simulink model "int_crit"  (Simulink 6.4)
settings: Solver=ode45  StartTime=0.0  StopTime=10.0  RelTol=1e-3
undefined symbols (not defined in the file or in its folder): q_de, q_du, q_u
settings Model: Creator=oravec  LastModifiedBy=oravec
settings OptimizationCC: InitFltsAndDblsToZero=off
settings DebuggingCC: SignalResolutionControl=UseLocalSettings  MultiTaskDSMMsg=error  MultiTaskCondExecSysMsg=error  StrictBusMsg=ErrorLevel1
settings HardwareCC: TargetHWDeviceType=32-bit Generic

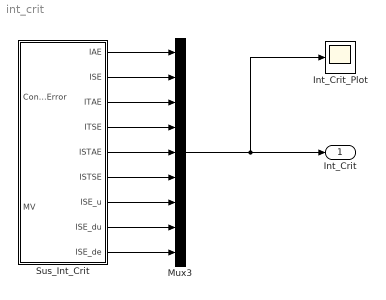
== system int_crit ==
  Int_Crit_Plot : Scope
  Mux3 : Mux  Inputs=9
  Sus_Int_Crit : Subsystem
  Int_Crit : Outport
  wires:
  Sus_Int_Crit/1(IAE) -> Mux3/1
  Sus_Int_Crit/3(ITAE) -> Mux3/3
  Sus_Int_Crit/4(ITSE) -> Mux3/4
  Sus_Int_Crit/5(ISTAE) -> Mux3/5
  Sus_Int_Crit/6(ISTSE) -> Mux3/6
  Sus_Int_Crit/7(ISE_u) -> Mux3/7
  Sus_Int_Crit/8(ISE_du) -> Mux3/8
  Sus_Int_Crit/9(ISE_de) -> Mux3/9
  Mux3/1 -> Int_Crit/1, Int_Crit_Plot/1
  Sus_Int_Crit/2(ISE) -> Mux3/2

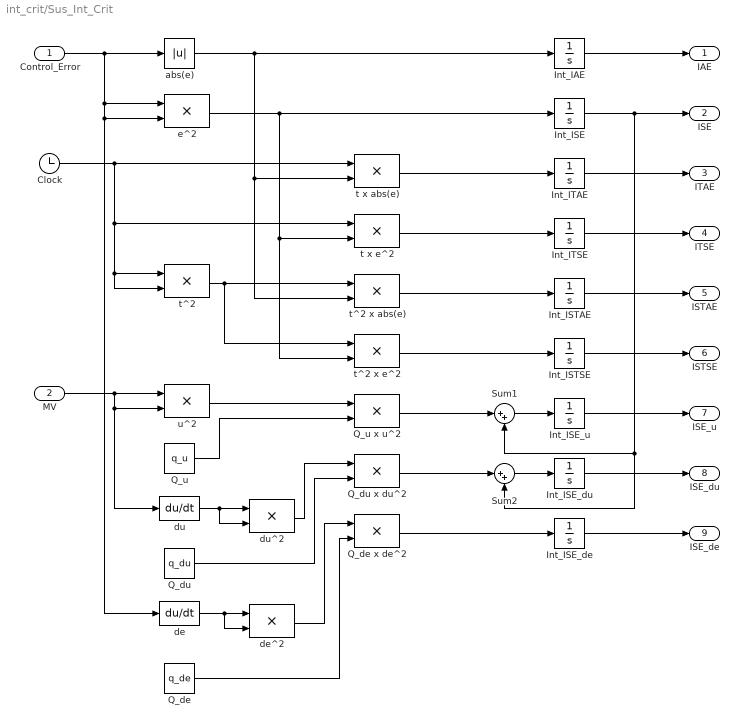
== system int_crit/Sus_Int_Crit ==
  Control_Error : Inport
  MV : Inport  Port=2
  Clock : Clock
      settings: Decimation=10
  Int_IAE : Integrator
  Int_ISE : Integrator
  Int_ISE_de : Integrator
  Int_ISE_du : Integrator
  Int_ISE_u : Integrator
  Int_ISTAE : Integrator
  Int_ISTSE : Integrator
  Int_ITAE : Integrator
  Int_ITSE : Integrator
  Q_de : Constant  Value=q_de
  Q_de x de^2 : Product  SaturateOnIntegerOverflow=on
  Q_du : Constant  Value=q_du
  Q_du x du^2 : Product  SaturateOnIntegerOverflow=on
  Q_u : Constant  Value=q_u
  Q_u x u^2 : Product  SaturateOnIntegerOverflow=on
  Sum1 : Sum  Inputs=|++  SaturateOnIntegerOverflow=on
  Sum2 : Sum  Inputs=|++  SaturateOnIntegerOverflow=on
  abs(e) : Abs  SaturateOnIntegerOverflow=on
  de : Derivative
  de^2 : Product  SaturateOnIntegerOverflow=on
  du : Derivative
  du^2 : Product  SaturateOnIntegerOverflow=on
  e^2 : Product  SaturateOnIntegerOverflow=on
  t x abs(e) : Product  SaturateOnIntegerOverflow=on
  t x e^2 : Product  SaturateOnIntegerOverflow=on
  t^2 : Product  SaturateOnIntegerOverflow=on
  t^2 x abs(e) : Product  SaturateOnIntegerOverflow=on
  t^2 x e^2 : Product  SaturateOnIntegerOverflow=on
  u^2 : Product  SaturateOnIntegerOverflow=on
  IAE : Outport
  ISE : Outport  Port=2
  ITAE : Outport  Port=3
  ITSE : Outport  Port=4
  ISTAE : Outport  Port=5
  ISTSE : Outport  Port=6
  ISE_u : Outport  Port=7
  ISE_du : Outport  Port=8
  ISE_de : Outport  Port=9
  wires:
  Control_Error/1 -> abs(e)/1, e^2/1, e^2/2, de/1
  abs(e)/1 -> Int_IAE/1, t x abs(e)/2, t^2 x abs(e)/2
  e^2/1 -> Int_ISE/1, t x e^2/2, t^2 x e^2/2
  Int_ISE/1 -> Sum1/2, Sum2/2, ISE/1
  t x abs(e)/1 -> Int_ITAE/1
  Clock/1 -> t x abs(e)/1, t x e^2/1, t^2/1, t^2/2
  t x e^2/1 -> Int_ITSE/1
  t^2/1 -> t^2 x abs(e)/1, t^2 x e^2/1
  t^2 x abs(e)/1 -> Int_ISTAE/1
  t^2 x e^2/1 -> Int_ISTSE/1
  Sum1/1 -> Int_ISE_u/1
  MV/1 -> u^2/1, u^2/2, du/1
  u^2/1 -> Q_u x u^2/1
  Q_u/1 -> Q_u x u^2/2
  Q_u x u^2/1 -> Sum1/1
  Sum2/1 -> Int_ISE_du/1
  du/1 -> du^2/1, du^2/2
  du^2/1 -> Q_du x du^2/1
  Q_du/1 -> Q_du x du^2/2
  Q_du x du^2/1 -> Sum2/1
  de/1 -> de^2/1, de^2/2
  de^2/1 -> Q_de x de^2/1
  Q_de/1 -> Q_de x de^2/2
  Q_de x de^2/1 -> Int_ISE_de/1
  Int_IAE/1 -> IAE/1
  Int_ITAE/1 -> ITAE/1
  Int_ITSE/1 -> ITSE/1
  Int_ISTAE/1 -> ISTAE/1
  Int_ISTSE/1 -> ISTSE/1
  Int_ISE_u/1 -> ISE_u/1
  Int_ISE_du/1 -> ISE_du/1
  Int_ISE_de/1 -> ISE_de/1
